simulink model "narx"  (R2019a)
settings: Solver=VariableStepAuto  StartTime=0.0  StopTime=10.0  RelTol=1e-3
libraries: neural x208
(part 2 of 5)

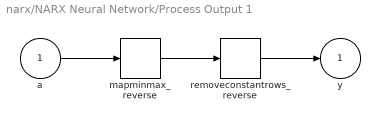
== system narx/NARX Neural Network/Process Output 1 ==
  a : Inport  PortDimensions=200  SampleTime=0.1
      mask Display: e = 0.06;c1 = [120 230 180]/255;c2 = ([120 230 180]+0)/(256+128);c3 = ([120 230 180]+128)/(256+128);patch([0 1 1 0],[0 0 1 1],c1);patch([0 1 1 1-e 1-e 0+e],[0 0 1 1-e 0+e 0+e],c2);patch([0 0 1 1-e 0+e 0+e],[0 1 1 1-e 1-e 0+e],c3);plot([0 1 1 0 0],[0 0 1 1 0]);
  mapminmax_reverse : neural/Processing Functions/mapminmax_reverse  xmin=[0.147625000000000006217248937901;0.433764527578450576061896981628;0.706630117733193729989693565585;0.966837544929993297770920435141;1.21497401801910775986925727921;1.45159950538667992248065274907;1.67724799863270335187337423122;1.89242871762729869544727989705;2.09762725966474672389949773788;2.29330669530856878779445651162;2.47990861340064228102164634038;2.65785411759261647191010524693;2.82754477664849979134942259407;2.98936353066295934510776532989;3.14367555524039143932668594061;3.29082908558495379480746123591;3.43115620236127627507016768504;3.5649735810993004037072751089;3.69258320683442597953671793221;3.81427305559568896597966158879;3.93031774427988267461842042394;4.04097915037818733452468222822;4.14650700295384666560494224541;4.24713944620454508793727654847;4.34310357688127268716016260441;4.43461595677647224533757253084;4.52188310143799654383656161372;4.60510194621174928641949009034;4.6844602906647381246330041904;4.76013722239145042891550474451;4.83230352115996986128720891429;4.90112204430985798353503923863;4.96674809427152830210161482682;5.02932976903649464617274134071;5.08900829636939899813796728267;5.145918352516025251475184632;5.20018836612654045126191704185;5.25194080807980778757837470039;5.30129246786283303549680567812;5.34835471712903931518212630181;5.3932337610301379626775997167;5.43603087788878802655290201074;5.47684264775289886273412776063;5.51576117034735879940399172483;5.55287427291504442905534233432;5.58826570841613445850271091331;5.62201534453301388083445999655;5.65419934390728862183550518239;5.68489033601565285636070257169;5.71415758107248006325562528218;5.74206712632901616899516739068;5.76868195512189352314180723624;5.79406212900732420223448571051;5.81826492330172406752808456076;5.84134495633464556618719143444;5.86335431270569973349893189152;5.88434266082362000815919600427;5.90435736499272234567570194486;5.9234435922997041856774558255;5.94164441454199110381750870147;5.95900090542765337175978856976;5.97555223326624851409860639251;5.99133574935975499187179593719;6.0063870722930774448400370602;6.02074016831433489471692155348;6.03442742798632902889721663087;6.04747973928217419370412244461;6.0599265572900344878348732891;6.07179597068428300588038837304;6.08311476511307525072425050894;6.09390848364539472470369219081;6.10420148441397270033803579281;6.11401699558417011104438643088;6.12337716777286544811431667767;6.13230312403564781220666191075;6.14081500753511200230150279822;6.14893202699783891773677169112;6.1566725000626352226618109853;6.16405389461786068494575374643;6.17109286822113034531867015176;6.17780530569034080912160789012;6.18420635495086568056422038353;6.19031046121980388363681413466;6.1961313996044333762824862788;6.20168230618842830637049701181;6.20697570767599504648615038604;6.21202354966082914700109540718;6.2168372235836741879211331252;6.22142759243933518575886409963;6.2258050152911446062375944166;6.22997937064821183383855895954;6.23396007875820679089429177111;6.23775612286598857281205710024;6.24137606948604872769692519796;6.24482808773452546802218421362;6.24811996776440814471698104171;6.25125913834553781356362378574;6.25425268362907615937729133293;6.25710735913427562593369657407;6.25982960699362855905292235548;6.26242557049079362485599631327;6.26490110792411769580212421715;6.26726180582702774302106263349;6.26951299157513464166413541534;6.27165974540849546770004963037;6.27370691189616813687734975247;6.2756591108689248059704368643;6.27752074784480473823577995063;6.27929602397102293309671949828;6.28098894550468056507952496759;6.28260333285366545652550485102;6.28414282919814848327177969622;6.28561090871212968522740993649;6.28701088440359345810293234535;6.28834591559095290591585580842;6.28961901503267206692271429347;6.29083305572614115419582958566;6.29199077739115786300772015238;6.29309479265263949088193839998;6.29414759293652004146224498982;6.29515155409213988946248719003;6.29610894175381297088733845158;6.29702191645367381767073311494;6.29789253849734009804706147406;6.29872277261339252873995064874 ...(+2390 chars)]  xmax=[3.69062500000000026645352591004;10.8441131894612627917240388342;17.6657529433298421395193145145;24.1709386232498317781391961034;30.3743504504776922203745925799;36.2899876346669998383731581271;41.9311999658175835747897508554;47.3107179406824656098251580261;52.440681491618661880238505546;57.3326673827142201389506226406;61.9977153350160605782548373099;66.4463529398154122418418410234;70.6886194162125036655197618529;74.7340882665739911772107006982;78.5918888810097939767729258165;82.2707271396238581928628263995;85.778905059031913538092339877;89.1243395274825189744660747238;92.3145801708606654756295029074;95.3568263898922481303088716231;98.2579436069970881817425834015;101.024478759454709120291227009;103.66267507384620216726034414;106.178486155113660061033442616;108.577589422031849153427174315;110.865398919411845213289780077;113.047077535949938464909791946;115.127548655293765023088781163;117.111507266618474432107177563;119.003430559786281150991271716;120.807588028999276730246492662;122.52805110774647801008541137;124.168702356788230645179282874;125.733244225912386582422186621;127.225207409234982947054959368;128.647958812900640168663812801;130.004709153163503287942148745;131.298520201995188472210429609;132.532311696570843650988535956;133.708867928225998866764712147;134.83084402575346416597312782;135.90077194721970954560674727;136.921066193822468903817934915;137.894029258683985972311347723;138.821856822876128489951952361;139.706642710403372120708809234;140.550383613325351461753598414;141.354983597682206664103432558;142.12225840039130275727075059;142.853939526811984706000657752;143.551678158225399783987086266;144.217048878047336302188341506;144.851553225183096174077945761;145.456623082543103464558953419;146.033623908366138266501366161;146.583857817642496002008556388;147.108566520590500203979900107;147.608934124818063082784647122;148.086089807492612635542172939;148.541110363549790918114013039;148.975022635691345840314170346;149.388805831656213740643579513;149.78339373399387568497331813;150.159676807326945890963543206;150.518504207858370591566199437;150.860685699658233716036193073;151.186993482054361948030418716;151.498163932250861307693412527;151.794899267107069817939191125;152.077869127826886597176780924;152.34771209113486634123546537;152.60503711034931484391563572;152.850424889604255440644919872;153.084429194321643308285274543;153.307578100891191752452868968;153.520375188377784070326015353;153.723300674945960508921416476;153.916812501565857473906362429;154.10134736544651445910858456;154.277321705528265738394111395;154.445132642258528221645974554;154.605158873771642902283929288;154.757761530495088209136156365;154.903284990110819308029022068;155.042057654710674796660896391;155.174392691899839746838551946;155.300588741520670055251684971;155.420930589591790749182109721;155.535689810983313918768544681;155.645125382278536108060507104;155.749484266205229232582496479;155.849001968955121810722630471;155.943903071649657476882566698;156.034401737151171118966885842;156.120702193363115384272532538;156.202999194110191183426650241;156.281478458638446227269014344;156.356317090726918195286998525;156.427683978356924399122362956;156.49574017484073351624829229;156.560639262269859273146721534;156.622527698102970816762535833;156.681545145675727326306514442;156.737824789378407785989111289;156.791493635212447088633780368;156.842672797404247830854728818;156.891477771723174328144523315;156.938018696120167305707582273;156.982400599275621289052651264;157.024723637617057647730689496;157.065083321341660393954953179;157.103570729953730733541306108;157.140272717803270552394678816;157.175272110089849775249604136;157.208647889773828865145333111;157.240475375816799896711017936;157.270826393153527078538900241;157.299769434778966115118237212;157.327369816316007700152113102;157.353689823413020576481358148;157.378788852303529210985288955;157.402723543845354470249731094;157.425547911341880080726696178;157.447313462433527320172288455;157.468069315334815883034025319 ...(+2394 chars)]  ymin=-1  ymax=1
      settings: SourceProductName=MATLAB Runtime - Deep Learning Toolbox  SourceProductBaseCode=Missing
  removeconstantrows_reverse : neural/Processing Functions/removeconstantrows_reverse  inputSize=201  constants=0  rearrange=[201 1 2 3 4 5 6 7 8 9 10 11 12 13 14 15 16 17 18 19 20 21 22 23 24 25 26 27 28 29 30 31 32 33 34 35 36 37 38 39 40 41 42 43 44 45 46 47 48 49 50 51 52 53 54 55 56 57 58 59 60 61 62 63 64 65 66 67 68 69 70 71 72 73 74 75 76 77 78 79 80 81 82 83 84 85 86 87 88 89 90 91 92 93 94 95 96 97 98 99 100 101 102 103 104 105 106 107 108 109 110 111 112 113 114 115 116 117 118 119 120 121 122 123 124 125 126 127 128 129 130 131 132 133 134 135 136 137 138 139 140 141 142 143 144 145 146 147 148 149 150 151 152 153 154 155 156 157 158 159 160 161 162 163 164 165 166 167 168 169 170 171 172 173 174 175 176 177 178 179 180 181 182 183 184 185 186 187 188 189 190 191 192 193 194 195 196 197 198 199 200]
      settings: SourceProductName=MATLAB Runtime - Deep Learning Toolbox  SourceProductBaseCode=Missing
  y : Outport  PortDimensions=201  SampleTime=0.1
      mask Display: e = 0.06;c1 = [120 230 180]/255;c2 = ([120 230 180]+0)/(256+128);c3 = ([120 230 180]+128)/(256+128);patch([0 1 1 0],[0 0 1 1],c1);patch([0 1 1 1-e 1-e 0+e],[0 0 1 1-e 0+e 0+e],c2);patch([0 0 1 1-e 0+e 0+e],[0 1 1 1-e 1-e 0+e],c3);plot([0 1 1 0 0],[0 0 1 1 0]);
  wires:
  a/1 -> mapminmax_reverse/1
  mapminmax_reverse/1 -> removeconstantrows_reverse/1
  removeconstantrows_reverse/1 -> y/1

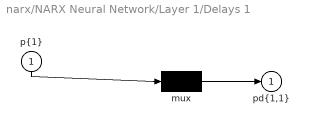
== system narx/NARX Neural Network/Layer 1/Delays 1 ==
  "p{1}" : Inport  PortDimensions=200  SampleTime=0.1
      mask Display: e = 0.06;c1 = [120 230 180]/255;c2 = ([120 230 180]+0)/(256+128);c3 = ([120 230 180]+128)/(256+128);patch([0 1 1 0],[0 0 1 1],c1);patch([0 1 1 1-e 1-e 0+e],[0 0 1 1-e 0+e 0+e],c2);patch([0 0 1 1-e 0+e 0+e],[0 1 1 1-e 1-e 0+e],c3);plot([0 1 1 0 0],[0 0 1 1 0]);
  mux : Mux  Inputs=1
      mask Display: e = 0.06;c1 = [120 150 230]/255;c2 = ([120 150 230]+0)/383;c3 = ([120 150 230]+128)/383;patch([0 1 1 0],[0 0 1 1],c1);patch([0 1 1 1-e 1-e 0+e],[0 0 1 1-e 0+e 0+e],c2);patch([0 0 1 1-e 0+e 0+e],[0 1 1 1-e 1-e 0+e],c3);plot([0 1 1 0 0],[0 0 1 1 0]);disp('Mux')
  "pd{1,1}" : Outport
      mask Display: e = 0.06;c1 = [120 230 180]/255;c2 = ([120 230 180]+0)/(256+128);c3 = ([120 230 180]+128)/(256+128);patch([0 1 1 0],[0 0 1 1],c1);patch([0 1 1 1-e 1-e 0+e],[0 0 1 1-e 0+e 0+e],c2);patch([0 0 1 1-e 0+e 0+e],[0 1 1 1-e 1-e 0+e],c3);plot([0 1 1 0 0],[0 0 1 1 0]);
  wires:
  "p{1}"/1 -> mux/1
  mux/1 -> "pd{1,1}"/1

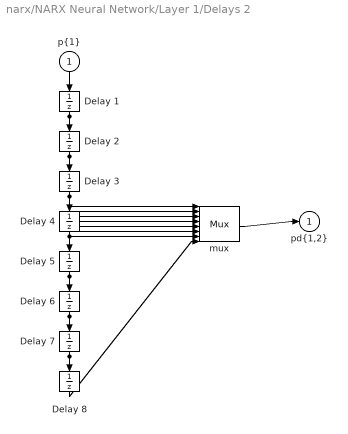
== system narx/NARX Neural Network/Layer 1/Delays 2 ==
  "p{1}" : Inport  PortDimensions=200  SampleTime=0.1
      mask Display: e = 0.06;c1 = [120 230 180]/255;c2 = ([120 230 180]+0)/(256+128);c3 = ([120 230 180]+128)/(256+128);patch([0 1 1 0],[0 0 1 1],c1);patch([0 1 1 1-e 1-e 0+e],[0 0 1 1-e 0+e 0+e],c2);patch([0 0 1 1-e 0+e 0+e],[0 1 1 1-e 1-e 0+e],c3);plot([0 1 1 0 0],[0 0 1 1 0]);
  Delay 1 : UnitDelay  InitialCondition=ai_layer_2_delayed_1  SampleTime=0.1
      mask Display: e = 0.06;c1 = [120 150 230]/255;c2 = ([120 150 230]+0)/383;c3 = ([120 150 230]+128)/383;patch([0 1 1 0],[0 0 1 1],c1);patch([0 1 1 1-e 1-e 0+e],[0 0 1 1-e 0+e 0+e],c2);patch([0 0 1 1-e 0+e 0+e],[0 1 1 1-e 1-e 0+e],c3);plot([0 1 1 0 0],[0 0 1 1 0]);disp('D')
  Delay 2 : UnitDelay  InitialCondition=ai_layer_2_delayed_2  SampleTime=0.1
      mask Display: e = 0.06;c1 = [120 150 230]/255;c2 = ([120 150 230]+0)/383;c3 = ([120 150 230]+128)/383;patch([0 1 1 0],[0 0 1 1],c1);patch([0 1 1 1-e 1-e 0+e],[0 0 1 1-e 0+e 0+e],c2);patch([0 0 1 1-e 0+e 0+e],[0 1 1 1-e 1-e 0+e],c3);plot([0 1 1 0 0],[0 0 1 1 0]);disp('D')
  Delay 3 : UnitDelay  InitialCondition=ai_layer_2_delayed_3  SampleTime=0.1
      mask Display: e = 0.06;c1 = [120 150 230]/255;c2 = ([120 150 230]+0)/383;c3 = ([120 150 230]+128)/383;patch([0 1 1 0],[0 0 1 1],c1);patch([0 1 1 1-e 1-e 0+e],[0 0 1 1-e 0+e 0+e],c2);patch([0 0 1 1-e 0+e 0+e],[0 1 1 1-e 1-e 0+e],c3);plot([0 1 1 0 0],[0 0 1 1 0]);disp('D')
  Delay 4 : UnitDelay  InitialCondition=ai_layer_2_delayed_4  SampleTime=0.1
      mask Display: e = 0.06;c1 = [120 150 230]/255;c2 = ([120 150 230]+0)/383;c3 = ([120 150 230]+128)/383;patch([0 1 1 0],[0 0 1 1],c1);patch([0 1 1 1-e 1-e 0+e],[0 0 1 1-e 0+e 0+e],c2);patch([0 0 1 1-e 0+e 0+e],[0 1 1 1-e 1-e 0+e],c3);plot([0 1 1 0 0],[0 0 1 1 0]);disp('D')
  Delay 5 : UnitDelay  InitialCondition=ai_layer_2_delayed_5  SampleTime=0.1
      mask Display: e = 0.06;c1 = [120 150 230]/255;c2 = ([120 150 230]+0)/383;c3 = ([120 150 230]+128)/383;patch([0 1 1 0],[0 0 1 1],c1);patch([0 1 1 1-e 1-e 0+e],[0 0 1 1-e 0+e 0+e],c2);patch([0 0 1 1-e 0+e 0+e],[0 1 1 1-e 1-e 0+e],c3);plot([0 1 1 0 0],[0 0 1 1 0]);disp('D')
  Delay 6 : UnitDelay  InitialCondition=ai_layer_2_delayed_6  SampleTime=0.1
      mask Display: e = 0.06;c1 = [120 150 230]/255;c2 = ([120 150 230]+0)/383;c3 = ([120 150 230]+128)/383;patch([0 1 1 0],[0 0 1 1],c1);patch([0 1 1 1-e 1-e 0+e],[0 0 1 1-e 0+e 0+e],c2);patch([0 0 1 1-e 0+e 0+e],[0 1 1 1-e 1-e 0+e],c3);plot([0 1 1 0 0],[0 0 1 1 0]);disp('D')
  Delay 7 : UnitDelay  InitialCondition=ai_layer_2_delayed_7  SampleTime=0.1
      mask Display: e = 0.06;c1 = [120 150 230]/255;c2 = ([120 150 230]+0)/383;c3 = ([120 150 230]+128)/383;patch([0 1 1 0],[0 0 1 1],c1);patch([0 1 1 1-e 1-e 0+e],[0 0 1 1-e 0+e 0+e],c2);patch([0 0 1 1-e 0+e 0+e],[0 1 1 1-e 1-e 0+e],c3);plot([0 1 1 0 0],[0 0 1 1 0]);disp('D')
  Delay 8 : UnitDelay  InitialCondition=ai_layer_2_delayed_8  SampleTime=0.1
      mask Display: e = 0.06;c1 = [120 150 230]/255;c2 = ([120 150 230]+0)/383;c3 = ([120 150 230]+128)/383;patch([0 1 1 0],[0 0 1 1],c1);patch([0 1 1 1-e 1-e 0+e],[0 0 1 1-e 0+e 0+e],c2);patch([0 0 1 1-e 0+e 0+e],[0 1 1 1-e 1-e 0+e],c3);plot([0 1 1 0 0],[0 0 1 1 0]);disp('D')
  mux : Mux  Inputs=8
      mask Display: e = 0.06;c1 = [120 150 230]/255;c2 = ([120 150 230]+0)/383;c3 = ([120 150 230]+128)/383;patch([0 1 1 0],[0 0 1 1],c1);patch([0 1 1 1-e 1-e 0+e],[0 0 1 1-e 0+e 0+e],c2);patch([0 0 1 1-e 0+e 0+e],[0 1 1 1-e 1-e 0+e],c3);plot([0 1 1 0 0],[0 0 1 1 0]);disp('Mux')
  "pd{1,2}" : Outport
      mask Display: e = 0.06;c1 = [120 230 180]/255;c2 = ([120 230 180]+0)/(256+128);c3 = ([120 230 180]+128)/(256+128);patch([0 1 1 0],[0 0 1 1],c1);patch([0 1 1 1-e 1-e 0+e],[0 0 1 1-e 0+e 0+e],c2);patch([0 0 1 1-e 0+e 0+e],[0 1 1 1-e 1-e 0+e],c3);plot([0 1 1 0 0],[0 0 1 1 0]);
  wires:
  "p{1}"/1 -> Delay 1/1
  Delay 1/1 -> Delay 2/1, mux/1
  Delay 2/1 -> Delay 3/1, mux/2
  Delay 3/1 -> Delay 4/1, mux/3
  Delay 4/1 -> Delay 5/1, mux/4
  Delay 5/1 -> Delay 6/1, mux/5
  Delay 6/1 -> Delay 7/1, mux/6
  Delay 7/1 -> Delay 8/1, mux/7
  Delay 8/1 -> mux/8
  mux/1 -> "pd{1,2}"/1

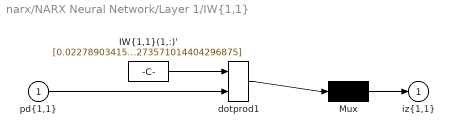
== system narx/NARX Neural Network/Layer 1/IW{1,1} ==
  "pd{1,1}" : Inport  PortDimensions=200  SampleTime=0.1
      mask Display: e = 0.06;c1 = [120 230 180]/255;c2 = ([120 230 180]+0)/(256+128);c3 = ([120 230 180]+128)/(256+128);patch([0 1 1 0],[0 0 1 1],c1);patch([0 1 1 1-e 1-e 0+e],[0 0 1 1-e 0+e 0+e],c2);patch([0 0 1 1-e 0+e 0+e],[0 1 1 1-e 1-e 0+e],c3);plot([0 1 1 0 0],[0 0 1 1 0]);
  "IW{1,1}(1,:)'" : Constant  Value=[0.0227890341577799172834151164579452597536146640777587890625;-0.03282051979613394288026739786801044829189777374267578125;-0.048950889123909623046326800022143288515508174896240234375;0.01477347843036840198405190704988854122348129749298095703125;0.0222483979174149422430861733346318942494690418243408203125;-0.022308691350345681569944389366355608217418193817138671875;0.0089852037524709611748807702724661794491112232208251953125;-0.020094993245088170474854649683038587681949138641357421875;0.0360833885146040478364426462576375342905521392822265625;-0.01448313747770632424483050471053502405993640422821044921875;0.023475012395247407681608819984830915927886962890625;0.016030857371492783502997525602040695957839488983154296875;0.053745380671429594798826911983269383199512958526611328125;-0.0332406271450272627898669952628551982343196868896484375;0.012016492673767829868491929801166406832635402679443359375;-0.046576194683090481329923449038687977008521556854248046875;0.0058935038184658450344244329244247637689113616943359375;0.040257575832464288778655969736064434982836246490478515625;-0.051473980902018483252202685207521426491439342498779296875;-0.01859869647621181787400246321340091526508331298828125;0.02467769217393434022511655712150968611240386962890625;0.041870433474262232220741708488276344723999500274658203125;0.00093752272554439007069826406137735830270685255527496337890625;0.057182686430705974289789850217857747338712215423583984375;-0.00729178798811491897524650340756124933250248432159423828125;-0.025661414306688841435732939544323016889393329620361328125;-0.002245191665610886400106238625085097737610340118408203125;-0.037790527003778724701721358769646030850708484649658203125;-0.038012326972067071728655918150252546183764934539794921875;-0.0255479000703650073467176895292141125537455081939697265625;0.0301182864660036915538388058166674454696476459503173828125;0.0132689397689374176392274051750064245425164699554443359375;0.054013563097918000643904434809883241541683673858642578125;0.031963359338559309275051845133930328302085399627685546875;0.00913371190846735785118237771484928089193999767303466796875;-0.00483382576920581182033931355590539169497787952423095703125;-0.0234165994434522260758679834680151543579995632171630859375;0.0295790641815350252574745582023751921951770782470703125;-0.045362783023670770476964975159717141650617122650146484375;-0.043947424052472545963343719677141052670776844024658203125;0.0275868174860606253651074126764797256328165531158447265625;-0.0157251479685343691083954098530739429406821727752685546875;0.0100183796755918021192943712094347574748098850250244140625;-0.0220729027642118935670367818602244369685649871826171875;0.0251709371019772261413027791832064394839107990264892578125;-0.01505386945353630323563010051657329313457012176513671875;0.025715162603324411005889515990929794497787952423095703125;0.0572467868454114292564582910927128978073596954345703125;-0.04657662778382831714196754546719603240489959716796875;-0.0027858537862141615100430858120716948178596794605255126953125;-0.0454260180333540819486159989537554793059825897216796875;0.0264794451296245410276686271799917449243366718292236328125;0.0477623504656990716110698258489719592034816741943359375;-0.046267497084006410645873330622634966857731342315673828125;0.003107303837649407797505407557991929934360086917877197265625;0.006829191633548063918024428886610621702857315540313720703125;0.0219214672563105179847742220999862183816730976104736328125;-0.021981881224548326103640505380099057219922542572021484375;0.01243782434155847431422881044227324309758841991424560546875;-0.0335017804917467076908366152565577067434787750244140625;0.0186880078255164949752042957697995007038116455078125;0.0234257274941735808837517396341354469768702983856201171875;-0.00375679293525191075608926638551565702073276042938232421875;-0.0381535247083915063370795905939303338527679443359375;-0.0080725465430638888852943324536681757308542728424072265625;0.01177463085358354359655219667502024094574153423309326171875 ...(+8113 chars)]
      mask Display: e = 0.06;c1 = [120 150 230]/255;c2 = ([120 150 230]+0)/383;c3 = ([120 150 230]+128)/383;patch([0 1 1 0],[0 0 1 1],c1);patch([0 1 1 1-e 1-e 0+e],[0 0 1 1-e 0+e 0+e],c2);patch([0 0 1 1-e 0+e 0+e],[0 1 1 1-e 1-e 0+e],c3);plot([0 1 1 0 0],[0 0 1 1 0]);disp('Weights');
  Mux : Mux  Inputs=1
      mask Display: e = 0.06;c1 = [120 150 230]/255;c2 = ([120 150 230]+0)/383;c3 = ([120 150 230]+128)/383;patch([0 1 1 0],[0 0 1 1],c1);patch([0 1 1 1-e 1-e 0+e],[0 0 1 1-e 0+e 0+e],c2);patch([0 0 1 1-e 0+e 0+e],[0 1 1 1-e 1-e 0+e],c3);plot([0 1 1 0 0],[0 0 1 1 0]);disp('Mux');
  dotprod1 : neural/Weight Functions/dotprod
      settings: SourceProductName=MATLAB Runtime - Deep Learning Toolbox  SourceProductBaseCode=Missing
  "iz{1,1}" : Outport
      mask Display: e = 0.06;c1 = [120 230 180]/255;c2 = ([120 230 180]+0)/(256+128);c3 = ([120 230 180]+128)/(256+128);patch([0 1 1 0],[0 0 1 1],c1);patch([0 1 1 1-e 1-e 0+e],[0 0 1 1-e 0+e 0+e],c2);patch([0 0 1 1-e 0+e 0+e],[0 1 1 1-e 1-e 0+e],c3);plot([0 1 1 0 0],[0 0 1 1 0]);
  wires:
  "IW{1,1}(1,:)'"/1 -> dotprod1/1
  "pd{1,1}"/1 -> dotprod1/2
  dotprod1/1 -> Mux/1
  Mux/1 -> "iz{1,1}"/1
